simulink model "SimulacionAleatoriosR16"  (Simulink 10.1)
settings: Solver=ode45  StartTime=0.0  StopTime=100  RelTol=1e-3  EnableMultiTasking=on
values from neighbouring files (symbols this model uses):
  net = train(net,P,T)    [AplicacionIdentificacion.m]    (also in AplicacionIdentificacionTest.m)
undefined symbols (not defined in the file or in its folder): sim
libraries: simulink x1
settings Model: Creator=Helbert  LastModifiedBy=leidy
settings DataIOCC: LimitDataPoints=on  SignalLoggingSaveFormat=ModelDataLogs
settings OptimizationCC: InitFltsAndDblsToZero=on
settings DebuggingCC: SaveWithParameterizedLinksMsg=none  SignalResolutionControl=TryResolveAllWithWarning  SolverPrmCheckMsg=warning  MultiTaskDSMMsg=warning  MultiTaskCondExecSysMsg=none
settings GRTTargetCC: TargetFcnLib=ansi_tfl_tmw.mat

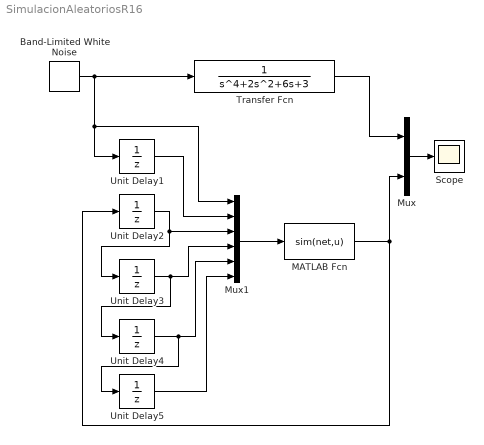
== system SimulacionAleatoriosR16 ==
  Band-Limited White Noise : simulink/Sources/Band-Limited White Noise  Cov=[0.1]  Ts=10  seed=[23341]
  MATLAB Fcn : MATLABFcn  MATLABFcn=sim(net,u)
  Mux : Mux  Inputs=2
  Mux1 : Mux  Inputs=6
  Scope : Scope
  Transfer Fcn : TransferFcn  Denominator=[1 0 2 6 3]
  Unit Delay{1..5} (5 alike) : UnitDelay  SampleTime=0.1  HasFrameUpgradeWarning=on
  wires:
  Mux/1 -> Scope/1
  Band-Limited White Noise/1 -> Unit Delay1/1, Mux1/1, Transfer Fcn/1
  MATLAB Fcn/1 -> Mux/2, Unit Delay2/1
  Unit Delay2/1 -> Unit Delay3/1, Mux1/3
  Mux1/1 -> MATLAB Fcn/1
  Unit Delay1/1 -> Mux1/2
  Unit Delay3/1 -> Unit Delay4/1, Mux1/4
  Transfer Fcn/1 -> Mux/1
  Unit Delay4/1 -> Unit Delay5/1, Mux1/5
  Unit Delay5/1 -> Mux1/6
